simulink model "friction_measurement"  (R2015b)
settings: Solver=ode45  StartTime=0.0  StopTime=10  RelTol=1e-3
undefined symbols (not defined in the file): AD622, Humusoft, Serial_Port, Standard_Devices
libraries: rtwinlib x2
settings Model: Creator=dave  LastModifiedBy=dave
settings DataIOCC: SaveFormat=StructureWithTime
settings HardwareCC: ProdWordSize=32  ProdHWDeviceType=Specified

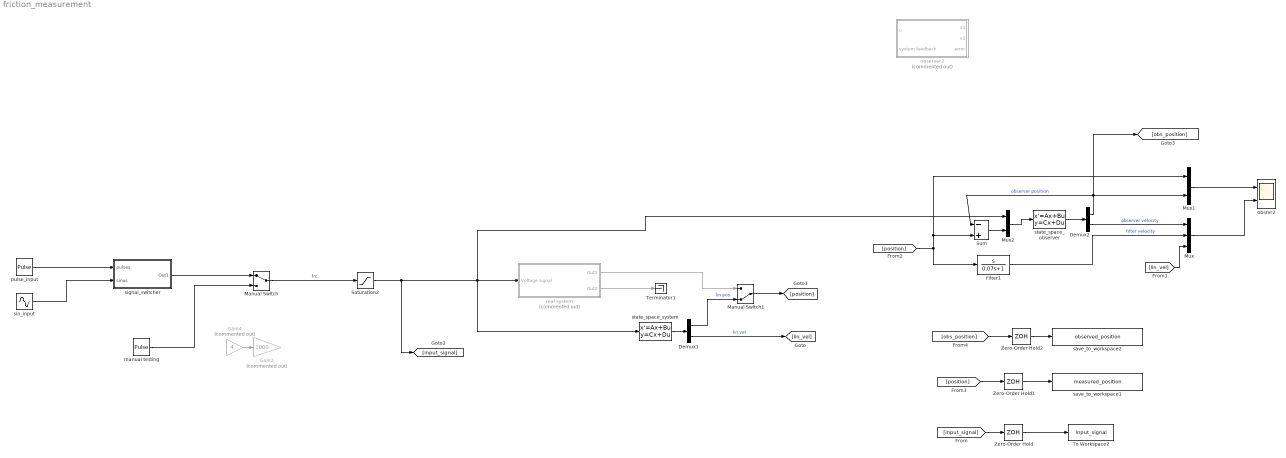
== system friction_measurement ==
  Demux1 : Demux  Outputs=2
  Demux2 : Demux  Outputs=2
  Filter1 : TransferFcn  Numerator=[1 0]  Denominator=[0.07 1]
  Gain2 : Gain  Commented=on  Gain=1000
  Gain4 : Gain  Commented=on  Gain=4
  Manual Switch : ManualSwitch
  Manual Switch1 : ManualSwitch  CurrentSetting=0
  Mux : Mux  Inputs=3
  Mux1 : Mux  Inputs=2
  Mux2 : Mux  Inputs=2
  Saturation2 : Saturate  UpperLimit=5  LowerLimit=-5
  Sum : Sum  Inputs=|-+
  Terminator1 : Terminator
  To Workspace2 : ToWorkspace  VariableName=input_signal  SaveFormat=Timeseries  SampleTime=-1
  Zero-Order Hold : ZeroOrderHold  SampleTime=0.01
  Zero-Order Hold1 : ZeroOrderHold  SampleTime=0.01
  Zero-Order Hold2 : ZeroOrderHold  SampleTime=0.01
  manual testing : DiscretePulseGenerator  PulseType=Time based  Period=6.5  PulseWidth=3  PhaseDelay=1
  observer2 : Subsystem  Commented=on
  obsrvr2 : Scope  NumInputPorts=2
  pulse_input : DiscretePulseGenerator  PulseType=Time based  Amplitude=4  Period=6.5  PulseWidth=3  PhaseDelay=1
  real system : Subsystem  Commented=on
  save_to_workspace1 : ToWorkspace  VariableName=measured_position  SaveFormat=Timeseries  SampleTime=-1
  save_to_workspace2 : ToWorkspace  VariableName=observed_position  SaveFormat=Timeseries  SampleTime=-1
  signal_switcher : Subsystem
  sin_input : Sin  Amplitude=5  Frequency=8  SampleTime=0
  state_space_observer : StateSpace  A=[0 1;0 -2.6]  B=[0 10;0.37037037037037 10]  C=[1 0;0 1]  D=[0 0;0 0]  X0=[0;0]
  state_space_system : StateSpace  A=[0 1;0 -2.6]  B=[0;0.37037037037037]  C=[1 0;0 1]  D=[0;0]  X0=[0;0]
  wires:
  Manual Switch/1 -> Saturation2/1  "frc"
  Gain4/1 -> Gain2/1
  Demux2/2 -> Mux/1  "observer velocity"
  state_space_system/1 -> Demux1/1
  Filter1/1 -> Mux/2  "filter velocity"
  Mux1/1 -> obsrvr2/1
  Mux/1 -> obsrvr2/2
  manual testing/1 -> Manual Switch/2
  Zero-Order Hold/1 -> To Workspace2/1
  Zero-Order Hold1/1 -> save_to_workspace1/1
  Demux1/1 -> Manual Switch1/2  "lin pos"
  real system/1(Out1) -> Manual Switch1/1
  real system/2(Out2) -> Terminator1/1
  pulse_input/1 -> signal_switcher/1(pulses)
  sin_input/1 -> signal_switcher/2(sinus)
  signal_switcher/1(Out1) -> Manual Switch/1
  Demux1/2 -> [lin_vel]  "lin vel"
  [lin_vel] -> Mux/3
  Manual Switch1/1 -> [position]
  [position] -> Zero-Order Hold1/1
  [input_signal] -> Zero-Order Hold/1
  Demux2/1 -> Mux1/2, [obs_position], Sum/1  "observer position"
  [obs_position] -> Zero-Order Hold2/1
  Zero-Order Hold2/1 -> save_to_workspace2/1
  Mux2/1 -> state_space_observer/1
  Sum/1 -> Mux2/2
  Saturation2/1 -> real system/1(Voltage signal), Mux2/1, state_space_system/1, [input_signal]
  [position] -> Sum/2, Mux1/1, Filter1/1
  state_space_observer/1 -> Demux2/1

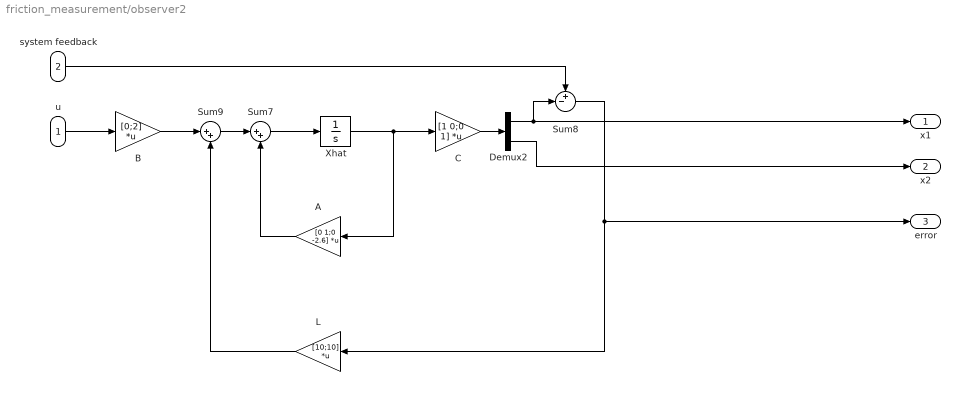
== system friction_measurement/observer2 ==
  u : Inport
  system feedback : Inport  Port=2
  A : Gain  Gain=[0 1;0 -2.6]  Multiplication=Matrix(K*u)
  B : Gain  Gain=[0;2]  Multiplication=Matrix(K*u)
  C : Gain  Gain=[1 0;0 1]  Multiplication=Matrix(K*u)
  Demux2 : Demux  Outputs=2
  L : Gain  Gain=[10;10]  Multiplication=Matrix(K*u)
  Sum7 : Sum  Inputs=|++
  Sum8 : Sum  Inputs=+-|
  Sum9 : Sum  Inputs=|++
  Xhat : Integrator  InitialCondition=[0 0]
  x1 : Outport
  x2 : Outport  Port=2
  error : Outport  Port=3
  wires:
  A/1 -> Sum7/2
  u/1 -> B/1
  Sum9/1 -> Sum7/1
  Xhat/1 -> A/1, C/1
  Sum8/1 -> L/1, error/1
  Sum7/1 -> Xhat/1
  system feedback/1 -> Sum8/1
  B/1 -> Sum9/1
  L/1 -> Sum9/2
  C/1 -> Demux2/1
  Demux2/1 -> Sum8/2, x1/1
  Demux2/2 -> x2/1

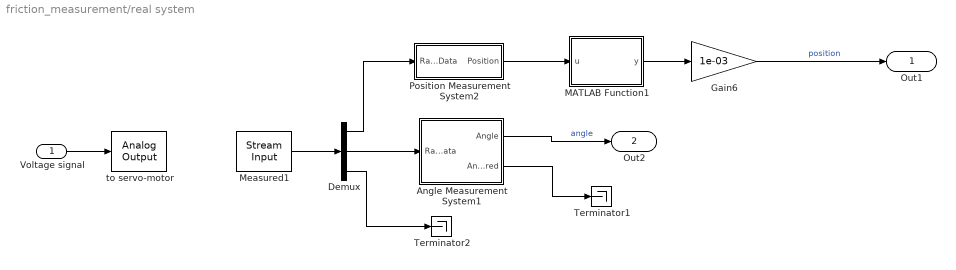
== system friction_measurement/real system ==
  Voltage signal : Inport
  Angle Measurement System1 : Subsystem
  Demux : Demux  Outputs=3
  Gain6 : Gain  Gain=1e-03
  MATLAB Function1 : MATLAB Function  TreatAsAtomicUnit=on
  Measured1 : rtwinlib/Stream Input  SampleTime=0.001  MaxMissedTicks=inf  ShowMissedTicks=off  YieldWhenWaiting=off  DrvName=Standard_Devices/Serial_Port  DrvAddress=1  DrvOptions=[115200 8 0 0 0 0 0 1]  DataTypes='3*double'  FormatString='%f%f%f'  Terminator={'\r\n'}  ShowReady=off  ShowError=off
      settings: AttributesFormatString=Standard Devices\nSerial Port [1h]
  Position Measurement System2 : Subsystem
  Terminator1 : Terminator
  Terminator2 : Terminator
  to servo-motor : rtwinlib/Analog Output  SampleTime=0.001  MaxMissedTicks=inf  ShowMissedTicks=off  YieldWhenWaiting=off  DrvName=Humusoft/AD622  DrvAddress=4294967295  DrvOptions=zeros(1,0)  Channels=2  RangeMode=1  VoltRange=1  InitialValue=0  FinalValue=0
      settings: AttributesFormatString=Humusoft\nAD622 [auto]
  Out1 : Outport
  Out2 : Outport  Port=2
  wires:
  Angle Measurement System1/2(Angle Filtered) -> Terminator1/1
  Angle Measurement System1/1(Angle) -> Out2/1  "angle"
  Measured1/1 -> Demux/1
  MATLAB Function1/1(y) -> Gain6/1
  Demux/3 -> Terminator2/1
  Demux/2 -> Angle Measurement System1/1(RawData)
  Position Measurement System2/1(Position) -> MATLAB Function1/1(u)
  Gain6/1 -> Out1/1  "position"
  Demux/1 -> Position Measurement System2/1(Raw Data)
  Voltage signal/1 -> to servo-motor/1

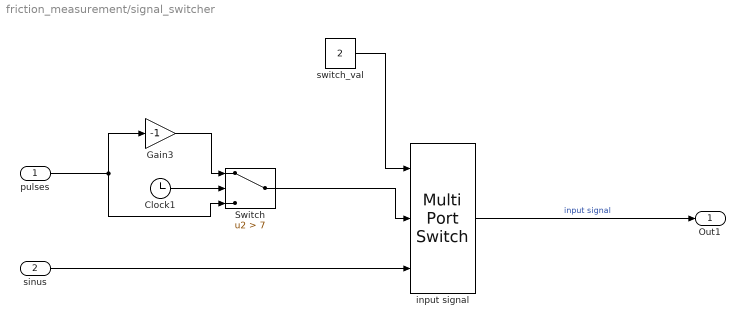
== system friction_measurement/signal_switcher ==
  pulses : Inport
  sinus : Inport  Port=2
  Clock1 : Clock
  Gain3 : Gain  Gain=-1
  Switch : Switch  Criteria=u2 > Threshold  Threshold=7
  input signal : MultiPortSwitch  Inputs=2
  switch_val : Constant  Value=2
  Out1 : Outport
  wires:
  pulses/1 -> Gain3/1, Switch/3
  input signal/1 -> Out1/1  "input signal"
  sinus/1 -> input signal/3
  Clock1/1 -> Switch/2
  Gain3/1 -> Switch/1
  switch_val/1 -> input signal/1
  Switch/1 -> input signal/2

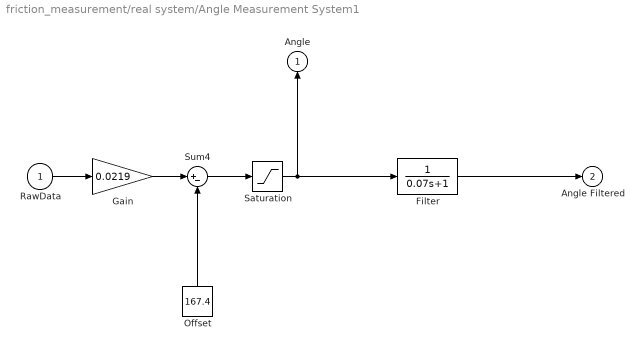
== system friction_measurement/real system/Angle Measurement System1 ==
  RawData : Inport
  Filter : TransferFcn  Denominator=[0.07 1]
  Gain : Gain  Gain=0.0219
  Offset : Constant  Value=167.4  SampleTime=-1
  Saturation : Saturate  UpperLimit=90  LowerLimit=-90
  Sum4 : Sum  Inputs=|+-
  Angle : Outport
  Angle Filtered : Outport  Port=2
  wires:
  RawData/1 -> Gain/1
  Sum4/1 -> Saturation/1
  Gain/1 -> Sum4/1
  Offset/1 -> Sum4/2
  Filter/1 -> Angle Filtered/1
  Saturation/1 -> Filter/1, Angle/1

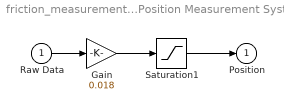
== system friction_measurement/real system/Position Measurement System2 ==
  Raw Data : Inport
  Gain : Gain  Gain=0.018
  Saturation1 : Saturate  UpperLimit=1600  LowerLimit=0
  Position : Outport
  wires:
  Raw Data/1 -> Gain/1
  Saturation1/1 -> Position/1
  Gain/1 -> Saturation1/1

== matlab function friction_measurement/real system/MATLAB Function1 ==
  data: u input; y output
function y = fcn(u)
%#codegen
if(0 <= u) && (u <= 600)
    y = u;
else
    y = u - 1179.576;
end
